simulink model "All_Simulations"  (R2022b)
settings: Solver=ode5  StartTime=0.0  StopTime=0.5  FixedStep=1e-4  RelTol=1e-3
undefined symbols (not defined in the file or in its folder): A_e, B_e, C_e, duration, effort, index, joint2, joint3, joint4, joint_name, K, L, model_name, open_manipulator
libraries: robotgazebolib x11
settings Model: Creator=User  LastModifiedBy=marin

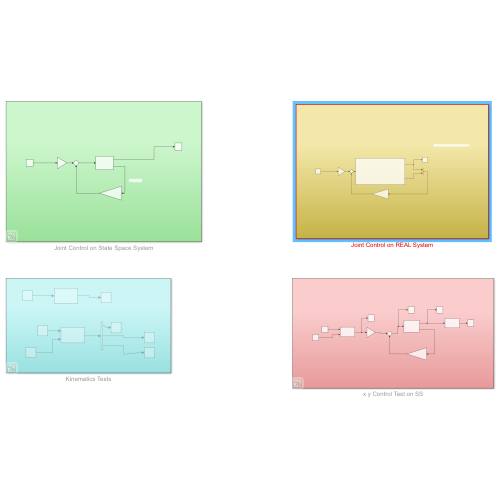
[thumbnail: Simulink's stored preview of the top-level diagram]
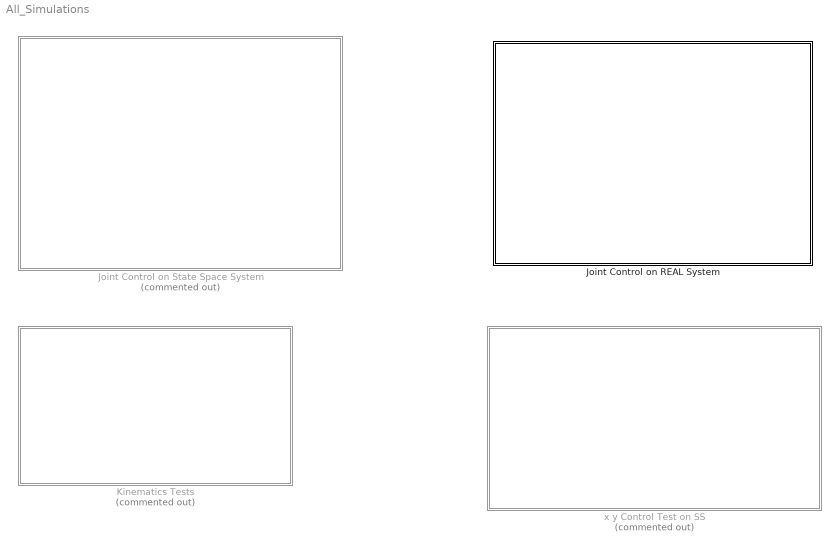
== system All_Simulations ==
  Joint Control on REAL System : Subsystem
  Joint Control on State Space System : Subsystem  Commented=on
  Kinematics Tests : Subsystem  Commented=on
  x y Control Test on SS : Subsystem  Commented=on

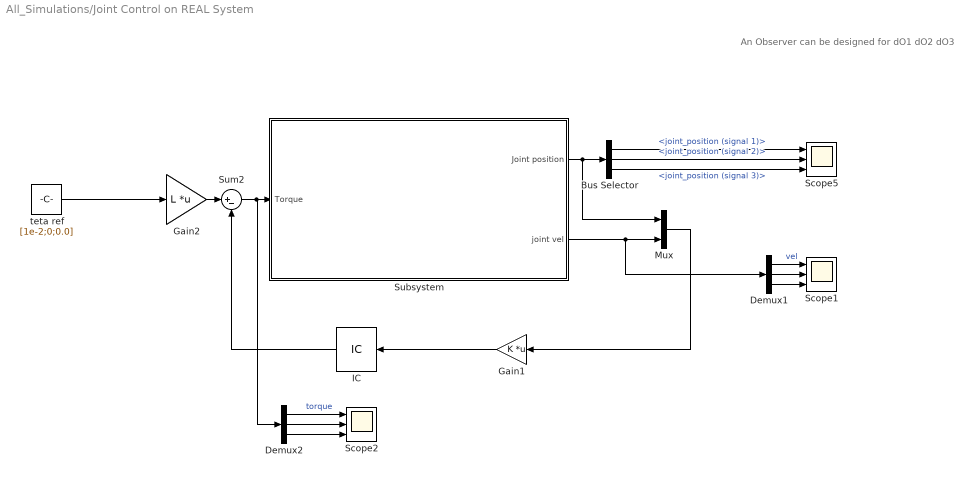
== system All_Simulations/Joint Control on REAL System ==
  note: An Observer can be designed for dO1 dO2 dO3
  Bus Selector : BusSelector  OutputSignals=joint_position (signal 1),joint_position (signal 2),joint_position (signal 3)
  Demux1 : Demux  Outputs=3
  Demux2 : Demux  Outputs=3
  Gain1 : Gain  Gain=K  Multiplication=Matrix(K*u)
  Gain2 : Gain  Gain=L  Multiplication=Matrix(K*u)
  IC : InitialCondition  Value=0
  Mux : Mux  Inputs=2
  Scope1 : Scope  NumInputPorts=3
  Scope2 : Scope  NumInputPorts=3
  Scope5 : Scope  NumInputPorts=3
  Subsystem : Subsystem
  Sum2 : Sum  Inputs=|+-
  teta ref : Constant  Value=[1e-2;0;0.0]
  wires:
  teta ref/1 -> Gain2/1
  Bus Selector/1 -> Scope5/1  "<joint_position (signal 1)>"
  Bus Selector/2 -> Scope5/2  "<joint_position (signal 2)>"
  Bus Selector/3 -> Scope5/3  "<joint_position (signal 3)>"
  Subsystem/2(joint vel) -> Demux1/1, Mux/2
  Gain2/1 -> Sum2/1
  Subsystem/1(Joint position) -> Mux/1, Bus Selector/1
  Mux/1 -> Gain1/1
  Gain1/1 -> IC/1
  IC/1 -> Sum2/2
  Demux1/1 -> Scope1/1  "vel"
  Demux1/2 -> Scope1/2
  Demux1/3 -> Scope1/3
  Demux2/1 -> Scope2/1  "torque"
  Demux2/2 -> Scope2/2
  Demux2/3 -> Scope2/3
  Sum2/1 -> Demux2/1, Subsystem/1(Torque)

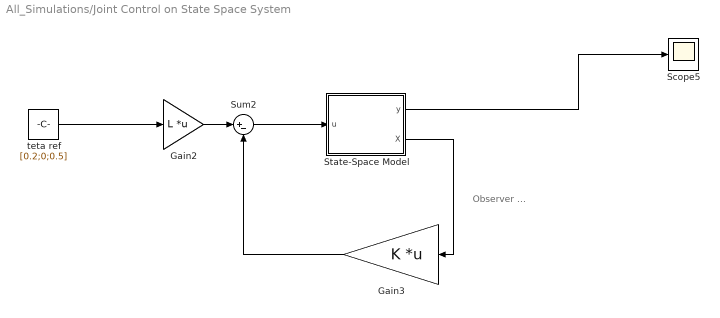
== system All_Simulations/Joint Control on State Space System ==
  note: Observer ...
  Gain2 : Gain  Gain=L  Multiplication=Matrix(K*u)
  Gain3 : Gain  Gain=K  Multiplication=Matrix(K*u)
  Scope5 : Scope
  State-Space Model : Subsystem
  Sum2 : Sum  Inputs=|+-
  teta ref : Constant  Value=[0.2;0;0.5]
  wires:
  State-Space Model/2(X) -> Gain3/1
  Sum2/1 -> State-Space Model/1(u)
  State-Space Model/1(y) -> Scope5/1
  Gain3/1 -> Sum2/2
  teta ref/1 -> Gain2/1
  Gain2/1 -> Sum2/1

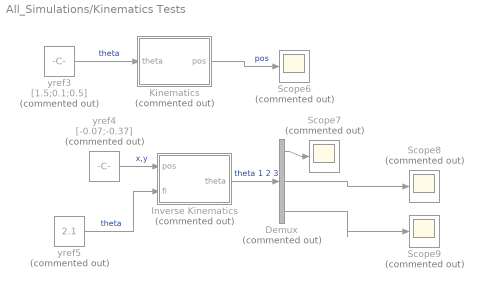
== system All_Simulations/Kinematics Tests ==
  Demux : Demux  Commented=on  Outputs=3
  Inverse Kinematics : MATLAB Function  Commented=on  TreatAsAtomicUnit=on
  Kinematics : MATLAB Function  Commented=on  TreatAsAtomicUnit=on
  Scope{6..9} (4 alike) : Scope  Commented=on
  yref3 : Constant  Commented=on  Value=[1.5;0.1;0.5]
  yref4 : Constant  Commented=on  Value=[-0.07;-0.37]
  yref5 : Constant  Commented=on  Value=2.1
  wires:
  Kinematics/1(pos) -> Scope6/1  "pos"
  yref4/1 -> Inverse Kinematics/1(pos)  "x,y"
  Demux/2 -> Scope8/1
  Inverse Kinematics/1(theta) -> Demux/1  "theta 1 2 3"
  Demux/3 -> Scope9/1
  yref3/1 -> Kinematics/1(theta)  "theta"
  yref5/1 -> Inverse Kinematics/2(fi)  "theta"
  Demux/1 -> Scope7/1

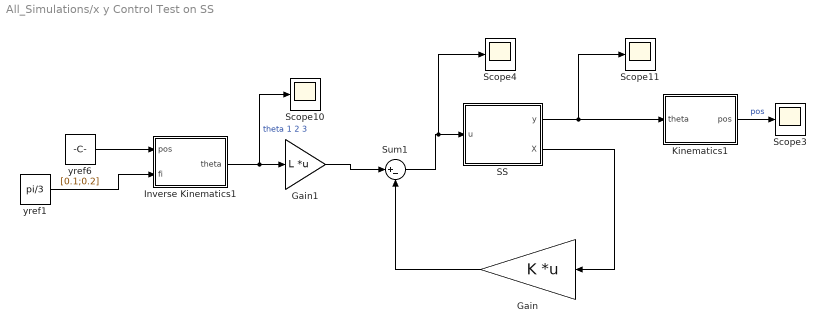
== system All_Simulations/x y Control Test on SS ==
  Gain : Gain  Gain=K  Multiplication=Matrix(K*u)
  Gain1 : Gain  Gain=L  Multiplication=Matrix(K*u)
  Inverse Kinematics1 : MATLAB Function  TreatAsAtomicUnit=on
  Kinematics1 : MATLAB Function  TreatAsAtomicUnit=on
  "SS " : Subsystem
  Scope{3..4,10..11} (4 alike) : Scope
  Sum1 : Sum  Inputs=|+-
  yref1 : Constant  Value=pi/3
  yref6 : Constant  Value=[0.1;0.2]
  wires:
  Inverse Kinematics1/1(theta) -> Scope10/1, Gain1/1  "theta 1 2 3"
  Sum1/1 -> Scope4/1, "SS "/1(u)
  Gain/1 -> Sum1/2
  "SS "/1(y) -> Scope11/1, Kinematics1/1(theta)
  yref1/1 -> Inverse Kinematics1/2(fi)
  Gain1/1 -> Sum1/1
  "SS "/2(X) -> Gain/1
  Kinematics1/1(pos) -> Scope3/1  "pos"
  yref6/1 -> Inverse Kinematics1/1(pos)

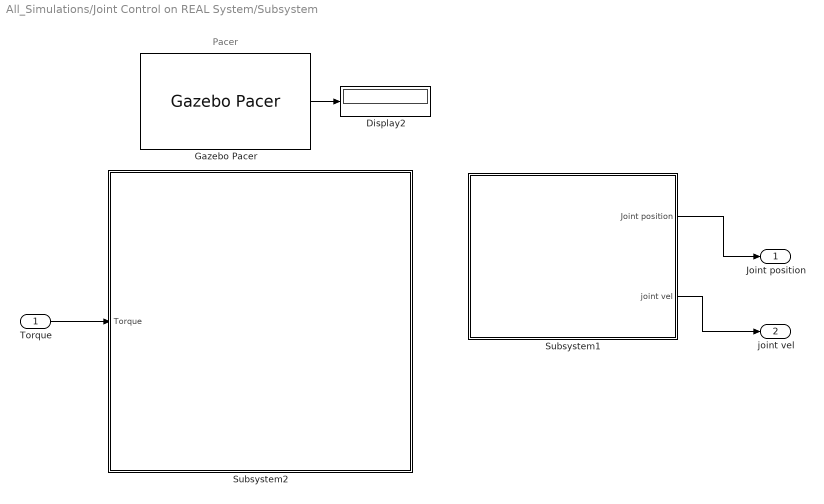
== system All_Simulations/Joint Control on REAL System/Subsystem ==
  note: Pacer
  Torque : Inport
  Display2 : Display
  Gazebo Pacer : robotgazebolib/Gazebo Pacer  ResetBehavior=Reset Gazebo simulation time and scene  SampleTime=0.01
  Subsystem1 : Subsystem
  Subsystem2 : Subsystem
  Joint position : Outport
  joint vel : Outport  Port=2
  wires:
  Gazebo Pacer/1 -> Display2/1
  Torque/1 -> Subsystem2/1(Torque)
  Subsystem1/1(Joint position) -> Joint position/1
  Subsystem1/2(joint vel) -> joint vel/1

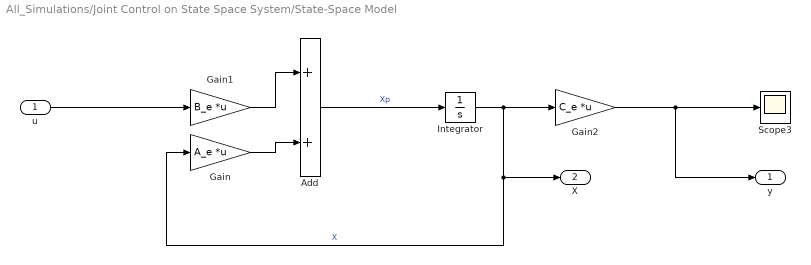
== system All_Simulations/Joint Control on State Space System/State-Space Model ==
  u : Inport
  Add : Sum
  Gain : Gain  Gain=A_e  Multiplication=Matrix(K*u)
  Gain1 : Gain  Gain=B_e  Multiplication=Matrix(K*u)
  Gain2 : Gain  Gain=C_e  Multiplication=Matrix(K*u)
  Integrator : Integrator
  Scope3 : Scope
  y : Outport
  X : Outport  Port=2
  wires:
  Integrator/1 -> Gain2/1, X/1, Gain/1  "X"
  Gain1/1 -> Add/1
  Add/1 -> Integrator/1  "Xp"
  Gain2/1 -> y/1, Scope3/1
  u/1 -> Gain1/1
  Gain/1 -> Add/2

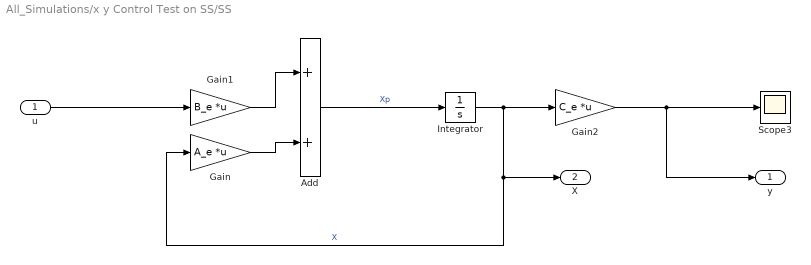
== system All_Simulations/x y Control Test on SS/SS  ==
  u : Inport
  Add : Sum
  Gain : Gain  Gain=A_e  Multiplication=Matrix(K*u)
  Gain1 : Gain  Gain=B_e  Multiplication=Matrix(K*u)
  Gain2 : Gain  Gain=C_e  Multiplication=Matrix(K*u)
  Integrator : Integrator
  Scope3 : Scope
  y : Outport
  X : Outport  Port=2
  wires:
  Integrator/1 -> Gain2/1, X/1, Gain/1  "X"
  Gain1/1 -> Add/1
  Add/1 -> Integrator/1  "Xp"
  Gain2/1 -> y/1, Scope3/1
  u/1 -> Gain1/1
  Gain/1 -> Add/2

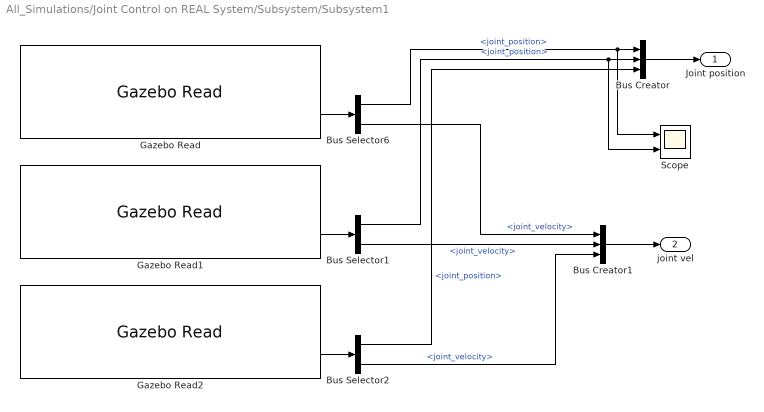
== system All_Simulations/Joint Control on REAL System/Subsystem/Subsystem1 ==
  Bus Creator : BusCreator  Inputs=3
  Bus Creator1 : BusCreator  Inputs=3
  Bus Selector1 : BusSelector  OutputSignals=joint_position,joint_velocity
  Bus Selector2 : BusSelector  OutputSignals=joint_position,joint_velocity
  Bus Selector6 : BusSelector  OutputSignals=joint_position,joint_velocity
  Gazebo Read : robotgazebolib/Gazebo Read  topicSource=From Gazebo  topic=/gazebo/ground_truth/joint_state/open_manipulator/joint2  messageType=gazebo_msgs/JointState  sampleTime=0.001  fixedAxisBusStatus=off  jointAxisCount=2
  Gazebo Read1 : robotgazebolib/Gazebo Read  topicSource=From Gazebo  topic=/gazebo/ground_truth/joint_state/open_manipulator/joint3  messageType=gazebo_msgs/JointState  sampleTime=0.001  fixedAxisBusStatus=off  jointAxisCount=2
  Gazebo Read2 : robotgazebolib/Gazebo Read  topicSource=From Gazebo  topic=/gazebo/ground_truth/joint_state/open_manipulator/joint4  messageType=gazebo_msgs/JointState  sampleTime=0.001  fixedAxisBusStatus=off  jointAxisCount=2
  Scope : Scope  NumInputPorts=2
  Joint position : Outport
  joint vel : Outport  Port=2
  wires:
  Gazebo Read/2 -> Bus Selector6/1
  Gazebo Read1/2 -> Bus Selector1/1
  Gazebo Read2/2 -> Bus Selector2/1
  Bus Selector6/2 -> Bus Creator1/1  "<joint_velocity>"
  Bus Selector1/2 -> Bus Creator1/2  "<joint_velocity>"
  Bus Selector2/2 -> Bus Creator1/3  "<joint_velocity>"
  Bus Creator1/1 -> joint vel/1
  Bus Creator/1 -> Joint position/1
  Bus Selector6/1 -> Scope/1, Bus Creator/1  "<joint_position>"
  Bus Selector1/1 -> Scope/2, Bus Creator/2  "<joint_position>"
  Bus Selector2/1 -> Bus Creator/3  "<joint_position>"

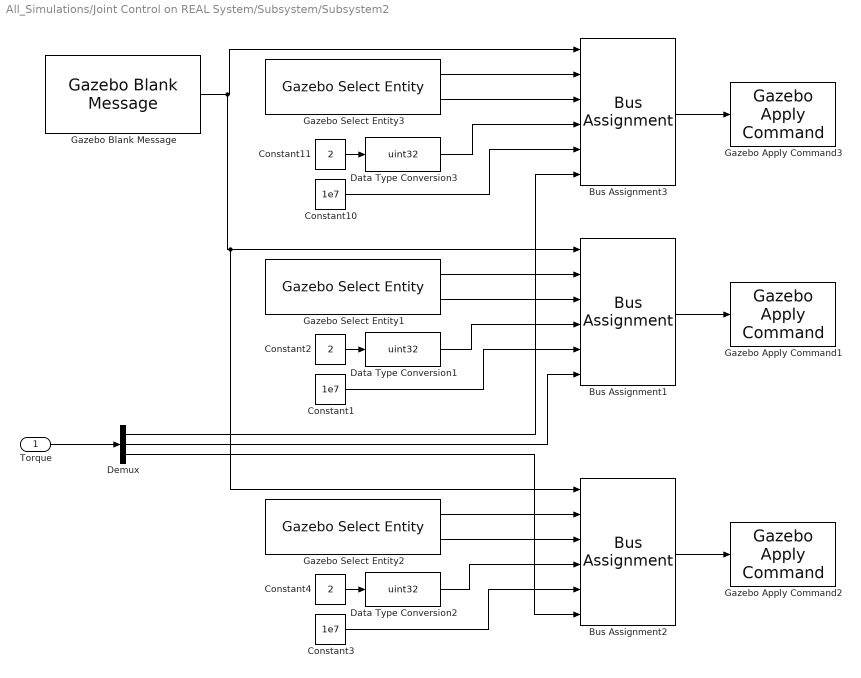
== system All_Simulations/Joint Control on REAL System/Subsystem/Subsystem2 ==
  Torque : Inport
  Bus Assignment1 : BusAssignment  AssignedSignals=model_name,joint_name,index,duration.nano_seconds,effort
  Bus Assignment2 : BusAssignment  AssignedSignals=model_name,joint_name,index,duration.nano_seconds,effort
  Bus Assignment3 : BusAssignment  AssignedSignals=model_name,joint_name,index,duration.nano_seconds,effort
  Constant1 : Constant  Value=1e7
  Constant10 : Constant  Value=1e7
  Constant11 : Constant  Value=2
  Constant2 : Constant  Value=2
  Constant3 : Constant  Value=1e7
  Constant4 : Constant  Value=2
  Data Type Conversion1 : DataTypeConversion  OutDataTypeStr=uint32  SaturateOnIntegerOverflow=off  RndMeth=Floor
  Data Type Conversion2 : DataTypeConversion  OutDataTypeStr=uint32  SaturateOnIntegerOverflow=off  RndMeth=Floor
  Data Type Conversion3 : DataTypeConversion  OutDataTypeStr=uint32  SaturateOnIntegerOverflow=off  RndMeth=Floor
  Demux : Demux  Outputs=3
  Gazebo Apply Command1 : robotgazebolib/Gazebo Apply Command  cmdType=ApplyJointTorque  sampleTime=0.01
  Gazebo Apply Command2 : robotgazebolib/Gazebo Apply Command  cmdType=ApplyJointTorque  sampleTime=0.01
  Gazebo Apply Command3 : robotgazebolib/Gazebo Apply Command  cmdType=ApplyJointTorque  sampleTime=0.01
  Gazebo Blank Message : robotgazebolib/Gazebo Blank Message  msgType=ApplyJointTorque  sampleTime=.001  busName='Gazebo_SL_Bus_gazebo_msgs_ApplyJointTorque'
  Gazebo Select Entity1 : robotgazebolib/Gazebo Select Entity  modelElemName=open_manipulator/joint3  outputArraySize=128  OutputLabel=Joint  SelectType=Joint
  Gazebo Select Entity2 : robotgazebolib/Gazebo Select Entity  modelElemName=open_manipulator/joint4  outputArraySize=128  OutputLabel=Joint  SelectType=Joint
  Gazebo Select Entity3 : robotgazebolib/Gazebo Select Entity  modelElemName=open_manipulator/joint2  outputArraySize=128  OutputLabel=Joint  SelectType=Joint
  wires:
  Constant11/1 -> Data Type Conversion3/1
  Gazebo Select Entity3/1 -> Bus Assignment3/2
  Constant10/1 -> Bus Assignment3/5
  Gazebo Select Entity3/2 -> Bus Assignment3/3
  Bus Assignment3/1 -> Gazebo Apply Command3/1
  Data Type Conversion3/1 -> Bus Assignment3/4
  Bus Assignment1/1 -> Gazebo Apply Command1/1
  Data Type Conversion1/1 -> Bus Assignment1/4
  Constant1/1 -> Bus Assignment1/5
  Gazebo Select Entity1/2 -> Bus Assignment1/3
  Constant2/1 -> Data Type Conversion1/1
  Bus Assignment2/1 -> Gazebo Apply Command2/1
  Data Type Conversion2/1 -> Bus Assignment2/4
  Constant3/1 -> Bus Assignment2/5
  Gazebo Select Entity2/2 -> Bus Assignment2/3
  Constant4/1 -> Data Type Conversion2/1
  Gazebo Select Entity2/1 -> Bus Assignment2/2
  Gazebo Select Entity1/1 -> Bus Assignment1/2
  Torque/1 -> Demux/1
  Gazebo Blank Message/1 -> Bus Assignment2/1, Bus Assignment1/1, Bus Assignment3/1
  Demux/1 -> Bus Assignment3/6
  Demux/2 -> Bus Assignment1/6
  Demux/3 -> Bus Assignment2/6

== matlab function All_Simulations/Kinematics Tests/Inverse Kinematics ==
  data: pos input; theta output; fi input
function theta= fcn(pos, fi)

% Masses des membres
m1 = 1.3850917e-01; % masse du membre inférieur
m2 = 1.3274562e-01; % masse du membre secondaire
m3 = 1.4327573e-01; % masse de la pince

% Longueurs des membres
l1 = 0.13; % longueur du membre inférieur
l2 = 0.124; % longueur du membre secondaire
l3 = 0.146; % longueur de la pince

x = pos(1);
y = pos(2);


xB = x - l3*cos(fi);
yB = x - l3*sin(fi);

theta2 = acos((xB^2+yB^2-l1^2-l2^2)/(2*l1*l2));

theta1 = asin(((l1+l2*cos(theta2 ))*yB - l2*sin(theta2 )*xB)/(xB^2 +yB^2));

theta3 = fi - theta1 - theta2;


theta = [theta1 ; theta2 ; theta3];

== matlab function All_Simulations/x y Control Test on SS/Kinematics1 ==
  data: theta input; pos output
function pos= fcn(theta)

% Masses des membres
m1 = 1.3850917e-01; % masse du membre inférieur
m2 = 1.3274562e-01; % masse du membre secondaire
m3 = 1.4327573e-01; % masse de la pince

% Longueurs des membres
l1 = 0.13; % longueur du membre inférieur
l2 = 0.124; % longueur du membre secondaire
l3 = 0.146; % longueur de la pince

theta1 = theta(1);
theta2 = theta(2);
theta3 = theta(3);

x = l1*cos(theta1) + l2*cos(theta1+theta2) + l3*cos(theta1+theta2+theta3);

y = l1*sin(theta1) + l2*sin(theta1+theta2) + l3*sin(theta1+theta2+theta3);


pos = [x ; y];

== matlab function All_Simulations/x y Control Test on SS/Inverse Kinematics1 ==
  data: pos input; theta output; fi input
function theta= fcn(pos, fi)

% Masses des membres
m1 = 1.3850917e-01; % masse du membre inférieur
m2 = 1.3274562e-01; % masse du membre secondaire
m3 = 1.4327573e-01; % masse de la pince

% Longueurs des membres
l1 = 0.13; % longueur du membre inférieur
l2 = 0.124; % longueur du membre secondaire
l3 = 0.146; % longueur de la pince

x = pos(1);
y = pos(2);


xB = x - l3*cos(fi);
yB = y - l3*sin(fi);

theta2 = acos((xB^2+yB^2-l1^2-l2^2)/(2*l1*l2));

theta1 = asin(((l1+l2*cos(theta2 ))*yB - l2*sin(theta2 )*xB)/(xB^2 +yB^2));

theta3 = fi - theta1 - theta2;


theta = [theta1 ; theta2 ; theta3];

== matlab function All_Simulations/Kinematics Tests/Kinematics ==
  data: theta input; pos output
function pos= fcn(theta)

% Masses des membres
m1 = 1.3850917e-01; % masse du membre inférieur
m2 = 1.3274562e-01; % masse du membre secondaire
m3 = 1.4327573e-01; % masse de la pince

% Longueurs des membres
l1 = 0.13; % longueur du membre inférieur
l2 = 0.124; % longueur du membre secondaire
l3 = 0.146; % longueur de la pince

theta1 = theta(1);
theta2 = theta(2);
theta3 = theta(3);

x = l1*cos(theta1) + l2*cos(theta1+theta2) + l3*cos(theta1+theta2+theta3);

y = l1*sin(theta1) + l2*sin(theta1+theta2) + l3*sin(theta1+theta2+theta3);


pos = [x ; y];
